simulink model "Motor_Quadcopter_Combined_Current"  (R2016b)
settings: Solver=VariableStepAuto  StartTime=0.0  StopTime=500  RelTol=1e-3
libraries: simulink x36
(part 3 of 5)

== system Motor_Quadcopter_Combined_Current/Nominal/Quadcopter_Arm1/Delta Motor ==
  Vab : Inport
  Vbc : Inport  Port=2
  Vca : Inport  Port=3
  1/Lm : Gain  Gain=100
  1/Lm1 : Gain  Gain=100
  1/Lm2 : Gain  Gain=100
  Add : Sum
  Add1 : Sum
  Constant : Constant  Value=5
  Constant1 : Constant  Value=5
  Constant2 : Constant  Value=5
  Divide : Product  Inputs=*/
  Gain : Gain  Gain=1/3
  Integrator : Integrator
  Integrator1 : Integrator
  Integrator2 : Integrator
  Mux : Mux  Inputs=1
  Product{,1..3} (4 alike) : Product
  motor current : Scope  NumInputPorts=3
  sum{,1..5} (6 alike) : Sum  Inputs=+-
  Out1 : Outport
  Out2 : Outport  Port=2
  wires:
  1/Lm2/1 -> Integrator2/1
  Integrator/1 -> Product1/1, sum5/2, sum3/1
  sum3/1 -> Mux/1, motor current/1  "i1"
  Vab/1 -> sum/1
  Product1/1 -> sum/2
  Integrator1/1 -> sum4/1, sum3/2, Product2/1
  sum1/1 -> 1/Lm1/1
  sum/1 -> 1/Lm/1
  1/Lm1/1 -> Integrator1/1
  Integrator2/1 -> sum5/1, sum4/2, Product3/1
  1/Lm/1 -> Integrator/1
  sum4/1 -> motor current/2  "i2"
  Product2/1 -> sum1/2
  Vca/1 -> sum2/1
  sum5/1 -> motor current/3  "i3"
  sum2/1 -> 1/Lm2/1
  Product3/1 -> sum2/2
  Vbc/1 -> sum1/1
  Mux/1 -> Out1/1
  Product/1 -> Divide/1
  Add/1 -> Divide/2
  Divide/1 -> Add1/1
  Constant/1 -> Add/1, Product/1, Product1/2
  Constant2/1 -> Add1/2, Product3/2
  Constant1/1 -> Add/2, Product/2, Product2/2
  Add1/1 -> Gain/1
  Gain/1 -> Out2/1

== system Motor_Quadcopter_Combined_Current/Nominal/Quadcopter_Arm1/Gate Driver ==
  Relational Operator{1..6} (6 alike) : RelationalOperator  Operator=>  OutDataTypeStr=boolean  RndMeth=Simplest
  Sawtooth{1..6} (6 alike) : SignalGenerator  WaveForm=sawtooth  Frequency=20
  Scope{1..6} (6 alike) : Scope  NumInputPorts=2
  Sine Wave (0 phase) : Sin  Frequency=2*pi  SampleTime=0.001
  Sine Wave (0.5 phase) : Sin  Frequency=2*pi  Phase=0.5*(2*pi)  SampleTime=0.001
  Sine Wave (0.5+1/3 phase) : Sin  Frequency=2*pi  Phase=(0.5 + 1/3)*(2*pi)  SampleTime=0.001
  Sine Wave (0.5+2/3 phase) : Sin  Frequency=2*pi  Phase=(2/3 + 0.5)*2*pi  SampleTime=0.001
  Sine Wave (1/3 phase) : Sin  Frequency=2*pi  Phase=(1/3)*(2*pi)  SampleTime=0.001
  Sine Wave (2/3 phase) : Sin  Frequency=2*pi  Phase=(2/3)*(2*pi)  SampleTime=0.001
  Switch {1..6} (6 alike) : Scope
  Switch 1 PWM : Outport
  Switch 2 PWM : Outport  Port=2
  Switch 3 PWM : Outport  Port=3
  Switch 4 PWM : Outport  Port=4
  Switch 5 PWM : Outport  Port=5
  Switch 6 PWM : Outport  Port=6
  wires:
  Relational Operator4/1 -> Switch 3 PWM/1, Switch 3/1
  Sine Wave (1/3 phase)/1 -> Scope2/1, Relational Operator3/1
  Relational Operator6/1 -> Switch 6 PWM/1, Switch 6/1
  Sine Wave (2/3 phase)/1 -> Scope4/1, Relational Operator4/1
  Sawtooth4/1 -> Scope4/2, Relational Operator4/2
  Sawtooth1/1 -> Scope1/2, Relational Operator1/2
  Relational Operator2/1 -> Switch 5 PWM/1, Switch 5/1
  Sine Wave (0.5+2/3 phase)/1 -> Scope6/1, Relational Operator6/1
  Sawtooth5/1 -> Scope5/2, Relational Operator5/2
  Relational Operator1/1 -> Switch 1 PWM/1, Switch 1/1
  Sawtooth6/1 -> Scope6/2, Relational Operator6/2
  Sine Wave (0 phase)/1 -> Scope1/1, Relational Operator1/1
  Sine Wave (0.5 phase)/1 -> Scope5/1, Relational Operator5/1
  Relational Operator3/1 -> Switch 2 PWM/1, Switch 2/1
  Sine Wave (0.5+1/3 phase)/1 -> Scope3/1, Relational Operator2/1
  Sawtooth2/1 -> Scope3/2, Relational Operator2/2
  Sawtooth3/1 -> Scope2/2, Relational Operator3/2
  Relational Operator5/1 -> Switch 4 PWM/1, Switch 4/1

== system Motor_Quadcopter_Combined_Current/Nominal/Quadcopter_Arm3/Delta Motor ==
  Vab : Inport
  Vbc : Inport  Port=2
  Vca : Inport  Port=3
  1/Lm : Gain  Gain=100
  1/Lm1 : Gain  Gain=100
  1/Lm2 : Gain  Gain=100
  Integrator : Integrator
  Integrator1 : Integrator
  Integrator2 : Integrator
  Rm : Gain  Gain=5
  Rm1 : Gain  Gain=5
  Rm2 : Gain  Gain=5
  motor current : Scope  NumInputPorts=3
  sum{,1..5} (6 alike) : Sum  Inputs=+-
  Out1 : Outport
  wires:
  1/Lm2/1 -> Integrator2/1
  Integrator/1 -> sum5/2, sum3/1, Rm/1
  sum3/1 -> Out1/1, motor current/1  "i1"
  Vab/1 -> sum/1
  Rm/1 -> sum/2
  Integrator1/1 -> sum4/1, sum3/2, Rm1/1
  sum1/1 -> 1/Lm1/1
  sum/1 -> 1/Lm/1
  1/Lm1/1 -> Integrator1/1
  Integrator2/1 -> sum5/1, sum4/2, Rm2/1
  1/Lm/1 -> Integrator/1
  sum4/1 -> motor current/2  "i2"
  Rm1/1 -> sum1/2
  Vca/1 -> sum2/1
  sum5/1 -> motor current/3  "i3"
  sum2/1 -> 1/Lm2/1
  Rm2/1 -> sum2/2
  Vbc/1 -> sum1/1

== system Motor_Quadcopter_Combined_Current/Nominal/Quadcopter_Arm3/Gate Driver ==
  Relational Operator{1..6} (6 alike) : RelationalOperator  Operator=>  OutDataTypeStr=boolean  RndMeth=Simplest
  Sawtooth{1..6} (6 alike) : SignalGenerator  WaveForm=sawtooth  Frequency=20
  Scope{1..6} (6 alike) : Scope  NumInputPorts=2
  Sine Wave (0 phase) : Sin  Frequency=2*pi  SampleTime=0.001
  Sine Wave (0.5 phase) : Sin  Frequency=2*pi  Phase=0.5*(2*pi)  SampleTime=0.001
  Sine Wave (0.5+1/3 phase) : Sin  Frequency=2*pi  Phase=(0.5 + 1/3)*(2*pi)  SampleTime=0.001
  Sine Wave (0.5+2/3 phase) : Sin  Frequency=2*pi  Phase=(2/3 + 0.5)*2*pi  SampleTime=0.001
  Sine Wave (1/3 phase) : Sin  Frequency=2*pi  Phase=(1/3)*(2*pi)  SampleTime=0.001
  Sine Wave (2/3 phase) : Sin  Frequency=2*pi  Phase=(2/3)*(2*pi)  SampleTime=0.001
  Switch {1..6} (6 alike) : Scope
  Switch 1 PWM : Outport
  Switch 2 PWM : Outport  Port=2
  Switch 3 PWM : Outport  Port=3
  Switch 4 PWM : Outport  Port=4
  Switch 5 PWM : Outport  Port=5
  Switch 6 PWM : Outport  Port=6
  wires:
  Relational Operator4/1 -> Switch 3 PWM/1, Switch 3/1
  Sine Wave (1/3 phase)/1 -> Scope2/1, Relational Operator3/1
  Relational Operator6/1 -> Switch 6 PWM/1, Switch 6/1
  Sine Wave (2/3 phase)/1 -> Scope4/1, Relational Operator4/1
  Sawtooth4/1 -> Scope4/2, Relational Operator4/2
  Sawtooth1/1 -> Scope1/2, Relational Operator1/2
  Relational Operator2/1 -> Switch 5 PWM/1, Switch 5/1
  Sine Wave (0.5+2/3 phase)/1 -> Scope6/1, Relational Operator6/1
  Sawtooth5/1 -> Scope5/2, Relational Operator5/2
  Relational Operator1/1 -> Switch 1 PWM/1, Switch 1/1
  Sawtooth6/1 -> Scope6/2, Relational Operator6/2
  Sine Wave (0 phase)/1 -> Scope1/1, Relational Operator1/1
  Sine Wave (0.5 phase)/1 -> Scope5/1, Relational Operator5/1
  Relational Operator3/1 -> Switch 2 PWM/1, Switch 2/1
  Sine Wave (0.5+1/3 phase)/1 -> Scope3/1, Relational Operator2/1
  Sawtooth2/1 -> Scope3/2, Relational Operator2/2
  Sawtooth3/1 -> Scope2/2, Relational Operator3/2
  Relational Operator5/1 -> Switch 4 PWM/1, Switch 4/1

== system Motor_Quadcopter_Combined_Current/Nominal/Quadcopter_Arm4/Delta Motor ==
  Vab : Inport
  Vbc : Inport  Port=2
  Vca : Inport  Port=3
  1/Lm : Gain  Gain=100
  1/Lm1 : Gain  Gain=100
  1/Lm2 : Gain  Gain=100
  Integrator : Integrator
  Integrator1 : Integrator
  Integrator2 : Integrator
  Rm : Gain  Gain=5
  Rm1 : Gain  Gain=5
  Rm2 : Gain  Gain=5
  motor current : Scope  NumInputPorts=3
  sum{,1..5} (6 alike) : Sum  Inputs=+-
  Out1 : Outport
  wires:
  1/Lm2/1 -> Integrator2/1
  Integrator/1 -> sum5/2, sum3/1, Rm/1
  sum3/1 -> Out1/1, motor current/1  "i1"
  Vab/1 -> sum/1
  Rm/1 -> sum/2
  Integrator1/1 -> sum4/1, sum3/2, Rm1/1
  sum1/1 -> 1/Lm1/1
  sum/1 -> 1/Lm/1
  1/Lm1/1 -> Integrator1/1
  Integrator2/1 -> sum5/1, sum4/2, Rm2/1
  1/Lm/1 -> Integrator/1
  sum4/1 -> motor current/2  "i2"
  Rm1/1 -> sum1/2
  Vca/1 -> sum2/1
  sum5/1 -> motor current/3  "i3"
  sum2/1 -> 1/Lm2/1
  Rm2/1 -> sum2/2
  Vbc/1 -> sum1/1

== system Motor_Quadcopter_Combined_Current/Nominal/Quadcopter_Arm4/Gate Driver ==
  Relational Operator{1..6} (6 alike) : RelationalOperator  Operator=>  OutDataTypeStr=boolean  RndMeth=Simplest
  Sawtooth{1..6} (6 alike) : SignalGenerator  WaveForm=sawtooth  Frequency=20
  Scope{1..6} (6 alike) : Scope  NumInputPorts=2
  Sine Wave (0 phase) : Sin  Frequency=2*pi  SampleTime=0.001
  Sine Wave (0.5 phase) : Sin  Frequency=2*pi  Phase=0.5*(2*pi)  SampleTime=0.001
  Sine Wave (0.5+1/3 phase) : Sin  Frequency=2*pi  Phase=(0.5 + 1/3)*(2*pi)  SampleTime=0.001
  Sine Wave (0.5+2/3 phase) : Sin  Frequency=2*pi  Phase=(2/3 + 0.5)*2*pi  SampleTime=0.001
  Sine Wave (1/3 phase) : Sin  Frequency=2*pi  Phase=(1/3)*(2*pi)  SampleTime=0.001
  Sine Wave (2/3 phase) : Sin  Frequency=2*pi  Phase=(2/3)*(2*pi)  SampleTime=0.001
  Switch {1..6} (6 alike) : Scope
  Switch 1 PWM : Outport
  Switch 2 PWM : Outport  Port=2
  Switch 3 PWM : Outport  Port=3
  Switch 4 PWM : Outport  Port=4
  Switch 5 PWM : Outport  Port=5
  Switch 6 PWM : Outport  Port=6
  wires:
  Relational Operator4/1 -> Switch 3 PWM/1, Switch 3/1
  Sine Wave (1/3 phase)/1 -> Scope2/1, Relational Operator3/1
  Relational Operator6/1 -> Switch 6 PWM/1, Switch 6/1
  Sine Wave (2/3 phase)/1 -> Scope4/1, Relational Operator4/1
  Sawtooth4/1 -> Scope4/2, Relational Operator4/2
  Sawtooth1/1 -> Scope1/2, Relational Operator1/2
  Relational Operator2/1 -> Switch 5 PWM/1, Switch 5/1
  Sine Wave (0.5+2/3 phase)/1 -> Scope6/1, Relational Operator6/1
  Sawtooth5/1 -> Scope5/2, Relational Operator5/2
  Relational Operator1/1 -> Switch 1 PWM/1, Switch 1/1
  Sawtooth6/1 -> Scope6/2, Relational Operator6/2
  Sine Wave (0 phase)/1 -> Scope1/1, Relational Operator1/1
  Sine Wave (0.5 phase)/1 -> Scope5/1, Relational Operator5/1
  Relational Operator3/1 -> Switch 2 PWM/1, Switch 2/1
  Sine Wave (0.5+1/3 phase)/1 -> Scope3/1, Relational Operator2/1
  Sawtooth2/1 -> Scope3/2, Relational Operator2/2
  Sawtooth3/1 -> Scope2/2, Relational Operator3/2
  Relational Operator5/1 -> Switch 4 PWM/1, Switch 4/1

== system Motor_Quadcopter_Combined_Current/Nominal/Quatcopter_Arm2/Delta Motor ==
  Vab : Inport
  Vbc : Inport  Port=2
  Vca : Inport  Port=3
  1/Lm : Gain  Gain=100
  1/Lm1 : Gain  Gain=100
  1/Lm2 : Gain  Gain=100
  Integrator : Integrator
  Integrator1 : Integrator
  Integrator2 : Integrator
  Mux : Mux  Inputs=1
  Rm : Gain  Gain=5
  Rm1 : Gain  Gain=5
  Rm2 : Gain  Gain=5
  motor current : Scope  NumInputPorts=3
  sum{,1..5} (6 alike) : Sum  Inputs=+-
  M2_Current : Outport
  wires:
  1/Lm2/1 -> Integrator2/1
  Integrator/1 -> sum5/2, sum3/1, Rm/1
  sum3/1 -> Mux/1, motor current/1  "i1"
  Vab/1 -> sum/1
  Rm/1 -> sum/2
  Integrator1/1 -> sum4/1, sum3/2, Rm1/1
  sum1/1 -> 1/Lm1/1
  sum/1 -> 1/Lm/1
  1/Lm1/1 -> Integrator1/1
  Integrator2/1 -> sum5/1, sum4/2, Rm2/1
  1/Lm/1 -> Integrator/1
  sum4/1 -> motor current/2  "i2"
  Rm1/1 -> sum1/2
  Vca/1 -> sum2/1
  sum5/1 -> motor current/3  "i3"
  sum2/1 -> 1/Lm2/1
  Rm2/1 -> sum2/2
  Vbc/1 -> sum1/1
  Mux/1 -> M2_Current/1

== system Motor_Quadcopter_Combined_Current/Nominal/Quatcopter_Arm2/Gate Driver ==
  Relational Operator{1..6} (6 alike) : RelationalOperator  Operator=>  OutDataTypeStr=boolean  RndMeth=Simplest
  Sawtooth{1..6} (6 alike) : SignalGenerator  WaveForm=sawtooth  Frequency=20
  Scope{1..6} (6 alike) : Scope  NumInputPorts=2
  Sine Wave (0 phase) : Sin  Frequency=2*pi  SampleTime=0.001
  Sine Wave (0.5 phase) : Sin  Frequency=2*pi  Phase=0.5*(2*pi)  SampleTime=0.001
  Sine Wave (0.5+1/3 phase) : Sin  Frequency=2*pi  Phase=(0.5 + 1/3)*(2*pi)  SampleTime=0.001
  Sine Wave (0.5+2/3 phase) : Sin  Frequency=2*pi  Phase=(2/3 + 0.5)*2*pi  SampleTime=0.001
  Sine Wave (1/3 phase) : Sin  Frequency=2*pi  Phase=(1/3)*(2*pi)  SampleTime=0.001
  Sine Wave (2/3 phase) : Sin  Frequency=2*pi  Phase=(2/3)*(2*pi)  SampleTime=0.001
  Switch {1..6} (6 alike) : Scope
  Switch 1 PWM : Outport
  Switch 2 PWM : Outport  Port=2
  Switch 3 PWM : Outport  Port=3
  Switch 4 PWM : Outport  Port=4
  Switch 5 PWM : Outport  Port=5
  Switch 6 PWM : Outport  Port=6
  wires:
  Relational Operator4/1 -> Switch 3 PWM/1, Switch 3/1
  Sine Wave (1/3 phase)/1 -> Scope2/1, Relational Operator3/1
  Relational Operator6/1 -> Switch 6 PWM/1, Switch 6/1
  Sine Wave (2/3 phase)/1 -> Scope4/1, Relational Operator4/1
  Sawtooth4/1 -> Scope4/2, Relational Operator4/2
  Sawtooth1/1 -> Scope1/2, Relational Operator1/2
  Relational Operator2/1 -> Switch 5 PWM/1, Switch 5/1
  Sine Wave (0.5+2/3 phase)/1 -> Scope6/1, Relational Operator6/1
  Sawtooth5/1 -> Scope5/2, Relational Operator5/2
  Relational Operator1/1 -> Switch 1 PWM/1, Switch 1/1
  Sawtooth6/1 -> Scope6/2, Relational Operator6/2
  Sine Wave (0 phase)/1 -> Scope1/1, Relational Operator1/1
  Sine Wave (0.5 phase)/1 -> Scope5/1, Relational Operator5/1
  Relational Operator3/1 -> Switch 2 PWM/1, Switch 2/1
  Sine Wave (0.5+1/3 phase)/1 -> Scope3/1, Relational Operator2/1
  Sawtooth2/1 -> Scope3/2, Relational Operator2/2
  Sawtooth3/1 -> Scope2/2, Relational Operator3/2
  Relational Operator5/1 -> Switch 4 PWM/1, Switch 4/1

== system Motor_Quadcopter_Combined_Current/PWM_Fault/Quadcopter_Arm1/Delta Motor ==
  Vab : Inport
  Vbc : Inport  Port=2
  Vca : Inport  Port=3
  1/Lm : Gain  Gain=100
  1/Lm1 : Gain  Gain=100
  1/Lm2 : Gain  Gain=100
  Add : Sum
  Add1 : Sum
  Constant : Constant  Value=5
  Constant1 : Constant  Value=5
  Constant2 : Constant  Value=5
  Divide : Product  Inputs=*/
  Gain : Gain  Gain=1/3
  Integrator : Integrator
  Integrator1 : Integrator
  Integrator2 : Integrator
  Mux : Mux  Inputs=1
  Product{,1..3} (4 alike) : Product
  motor current : Scope  NumInputPorts=3
  sum{,1..5} (6 alike) : Sum  Inputs=+-
  Out1 : Outport
  Out2 : Outport  Port=2
  wires:
  1/Lm2/1 -> Integrator2/1
  Integrator/1 -> Product1/1, sum5/2, sum3/1
  sum3/1 -> Mux/1, motor current/1  "i1"
  Vab/1 -> sum/1
  Product1/1 -> sum/2
  Integrator1/1 -> sum4/1, sum3/2, Product2/1
  sum1/1 -> 1/Lm1/1
  sum/1 -> 1/Lm/1
  1/Lm1/1 -> Integrator1/1
  Integrator2/1 -> sum5/1, sum4/2, Product3/1
  1/Lm/1 -> Integrator/1
  sum4/1 -> motor current/2  "i2"
  Product2/1 -> sum1/2
  Vca/1 -> sum2/1
  sum5/1 -> motor current/3  "i3"
  sum2/1 -> 1/Lm2/1
  Product3/1 -> sum2/2
  Vbc/1 -> sum1/1
  Mux/1 -> Out1/1
  Product/1 -> Divide/1
  Add/1 -> Divide/2
  Divide/1 -> Add1/1
  Constant/1 -> Add/1, Product/1, Product1/2
  Constant2/1 -> Add1/2, Product3/2
  Constant1/1 -> Add/2, Product/2, Product2/2
  Add1/1 -> Gain/1
  Gain/1 -> Out2/1

== system Motor_Quadcopter_Combined_Current/PWM_Fault/Quadcopter_Arm1/Gate Driver ==
  Relational Operator{1..6} (6 alike) : RelationalOperator  Operator=>  OutDataTypeStr=boolean  RndMeth=Simplest
  Sawtooth{1..6} (6 alike) : SignalGenerator  WaveForm=sawtooth  Frequency=20
  Scope{1..6} (6 alike) : Scope  NumInputPorts=2
  Sine Wave (0 phase) : Sin  Frequency=2*pi  SampleTime=0.001
  Sine Wave (0.5 phase) : Sin  Frequency=2*pi  Phase=0.5*(2*pi)  SampleTime=0.001
  Sine Wave (0.5+1/3 phase) : Sin  Frequency=2*pi  Phase=(0.5 + 1/3)*(2*pi)  SampleTime=0.001
  Sine Wave (0.5+2/3 phase) : Sin  Frequency=2*pi  Phase=(2/3 + 0.5)*2*pi  SampleTime=0.001
  Sine Wave (1/3 phase) : Sin  Frequency=2*pi  Phase=(1/3)*(2*pi)  SampleTime=0.001
  Sine Wave (2/3 phase) : Sin  Frequency=2*pi  Phase=(2/3)*(2*pi)  SampleTime=0.001
  Switch {1..6} (6 alike) : Scope
  Switch 1 PWM : Outport
  Switch 2 PWM : Outport  Port=2
  Switch 3 PWM : Outport  Port=3
  Switch 4 PWM : Outport  Port=4
  Switch 5 PWM : Outport  Port=5
  Switch 6 PWM : Outport  Port=6
  wires:
  Relational Operator4/1 -> Switch 3 PWM/1, Switch 3/1
  Sine Wave (1/3 phase)/1 -> Scope2/1, Relational Operator3/1
  Relational Operator6/1 -> Switch 6 PWM/1, Switch 6/1
  Sine Wave (2/3 phase)/1 -> Scope4/1, Relational Operator4/1
  Sawtooth4/1 -> Scope4/2, Relational Operator4/2
  Sawtooth1/1 -> Scope1/2, Relational Operator1/2
  Relational Operator2/1 -> Switch 5 PWM/1, Switch 5/1
  Sine Wave (0.5+2/3 phase)/1 -> Scope6/1, Relational Operator6/1
  Sawtooth5/1 -> Scope5/2, Relational Operator5/2
  Relational Operator1/1 -> Switch 1 PWM/1, Switch 1/1
  Sawtooth6/1 -> Scope6/2, Relational Operator6/2
  Sine Wave (0 phase)/1 -> Scope1/1, Relational Operator1/1
  Sine Wave (0.5 phase)/1 -> Scope5/1, Relational Operator5/1
  Relational Operator3/1 -> Switch 2 PWM/1, Switch 2/1
  Sine Wave (0.5+1/3 phase)/1 -> Scope3/1, Relational Operator2/1
  Sawtooth2/1 -> Scope3/2, Relational Operator2/2
  Sawtooth3/1 -> Scope2/2, Relational Operator3/2
  Relational Operator5/1 -> Switch 4 PWM/1, Switch 4/1

== system Motor_Quadcopter_Combined_Current/PWM_Fault/Quadcopter_Arm3/Delta Motor ==
  Vab : Inport
  Vbc : Inport  Port=2
  Vca : Inport  Port=3
  1/Lm : Gain  Gain=100
  1/Lm1 : Gain  Gain=100
  1/Lm2 : Gain  Gain=100
  Integrator : Integrator
  Integrator1 : Integrator
  Integrator2 : Integrator
  Rm : Gain  Gain=5
  Rm1 : Gain  Gain=5
  Rm2 : Gain  Gain=5
  motor current : Scope  NumInputPorts=3
  sum{,1..5} (6 alike) : Sum  Inputs=+-
  Out1 : Outport
  wires:
  1/Lm2/1 -> Integrator2/1
  Integrator/1 -> sum5/2, sum3/1, Rm/1
  sum3/1 -> Out1/1, motor current/1  "i1"
  Vab/1 -> sum/1
  Rm/1 -> sum/2
  Integrator1/1 -> sum4/1, sum3/2, Rm1/1
  sum1/1 -> 1/Lm1/1
  sum/1 -> 1/Lm/1
  1/Lm1/1 -> Integrator1/1
  Integrator2/1 -> sum5/1, sum4/2, Rm2/1
  1/Lm/1 -> Integrator/1
  sum4/1 -> motor current/2  "i2"
  Rm1/1 -> sum1/2
  Vca/1 -> sum2/1
  sum5/1 -> motor current/3  "i3"
  sum2/1 -> 1/Lm2/1
  Rm2/1 -> sum2/2
  Vbc/1 -> sum1/1

== system Motor_Quadcopter_Combined_Current/PWM_Fault/Quadcopter_Arm3/Gate Driver ==
  Relational Operator{1..6} (6 alike) : RelationalOperator  Operator=>  OutDataTypeStr=boolean  RndMeth=Simplest
  Sawtooth{1..6} (6 alike) : SignalGenerator  WaveForm=sawtooth  Frequency=20
  Scope{1..6} (6 alike) : Scope  NumInputPorts=2
  Sine Wave (0 phase) : Sin  Frequency=2*pi  SampleTime=0.001
  Sine Wave (0.5 phase) : Sin  Frequency=2*pi  Phase=0.5*(2*pi)  SampleTime=0.001
  Sine Wave (0.5+1/3 phase) : Sin  Frequency=2*pi  Phase=(0.5 + 1/3)*(2*pi)  SampleTime=0.001
  Sine Wave (0.5+2/3 phase) : Sin  Frequency=2*pi  Phase=(2/3 + 0.5)*2*pi  SampleTime=0.001
  Sine Wave (1/3 phase) : Sin  Frequency=2*pi  Phase=(1/3)*(2*pi)  SampleTime=0.001
  Sine Wave (2/3 phase) : Sin  Frequency=2*pi  Phase=(2/3)*(2*pi)  SampleTime=0.001
  Switch {1..6} (6 alike) : Scope
  Switch 1 PWM : Outport
  Switch 2 PWM : Outport  Port=2
  Switch 3 PWM : Outport  Port=3
  Switch 4 PWM : Outport  Port=4
  Switch 5 PWM : Outport  Port=5
  Switch 6 PWM : Outport  Port=6
  wires:
  Relational Operator4/1 -> Switch 3 PWM/1, Switch 3/1
  Sine Wave (1/3 phase)/1 -> Scope2/1, Relational Operator3/1
  Relational Operator6/1 -> Switch 6 PWM/1, Switch 6/1
  Sine Wave (2/3 phase)/1 -> Scope4/1, Relational Operator4/1
  Sawtooth4/1 -> Scope4/2, Relational Operator4/2
  Sawtooth1/1 -> Scope1/2, Relational Operator1/2
  Relational Operator2/1 -> Switch 5 PWM/1, Switch 5/1
  Sine Wave (0.5+2/3 phase)/1 -> Scope6/1, Relational Operator6/1
  Sawtooth5/1 -> Scope5/2, Relational Operator5/2
  Relational Operator1/1 -> Switch 1 PWM/1, Switch 1/1
  Sawtooth6/1 -> Scope6/2, Relational Operator6/2
  Sine Wave (0 phase)/1 -> Scope1/1, Relational Operator1/1
  Sine Wave (0.5 phase)/1 -> Scope5/1, Relational Operator5/1
  Relational Operator3/1 -> Switch 2 PWM/1, Switch 2/1
  Sine Wave (0.5+1/3 phase)/1 -> Scope3/1, Relational Operator2/1
  Sawtooth2/1 -> Scope3/2, Relational Operator2/2
  Sawtooth3/1 -> Scope2/2, Relational Operator3/2
  Relational Operator5/1 -> Switch 4 PWM/1, Switch 4/1

== system Motor_Quadcopter_Combined_Current/PWM_Fault/Quadcopter_Arm4/Delta Motor ==
  Vab : Inport
  Vbc : Inport  Port=2
  Vca : Inport  Port=3
  1/Lm : Gain  Gain=100
  1/Lm1 : Gain  Gain=100
  1/Lm2 : Gain  Gain=100
  Integrator : Integrator
  Integrator1 : Integrator
  Integrator2 : Integrator
  Rm : Gain  Gain=5
  Rm1 : Gain  Gain=5
  Rm2 : Gain  Gain=5
  motor current : Scope  NumInputPorts=3
  sum{,1..5} (6 alike) : Sum  Inputs=+-
  Out1 : Outport
  wires:
  1/Lm2/1 -> Integrator2/1
  Integrator/1 -> sum5/2, sum3/1, Rm/1
  sum3/1 -> Out1/1, motor current/1  "i1"
  Vab/1 -> sum/1
  Rm/1 -> sum/2
  Integrator1/1 -> sum4/1, sum3/2, Rm1/1
  sum1/1 -> 1/Lm1/1
  sum/1 -> 1/Lm/1
  1/Lm1/1 -> Integrator1/1
  Integrator2/1 -> sum5/1, sum4/2, Rm2/1
  1/Lm/1 -> Integrator/1
  sum4/1 -> motor current/2  "i2"
  Rm1/1 -> sum1/2
  Vca/1 -> sum2/1
  sum5/1 -> motor current/3  "i3"
  sum2/1 -> 1/Lm2/1
  Rm2/1 -> sum2/2
  Vbc/1 -> sum1/1

== system Motor_Quadcopter_Combined_Current/PWM_Fault/Quadcopter_Arm4/Gate Driver ==
  Relational Operator{1..6} (6 alike) : RelationalOperator  Operator=>  OutDataTypeStr=boolean  RndMeth=Simplest
  Sawtooth{1..6} (6 alike) : SignalGenerator  WaveForm=sawtooth  Frequency=20
  Scope{1..6} (6 alike) : Scope  NumInputPorts=2
  Sine Wave (0 phase) : Sin  Frequency=2*pi  SampleTime=0.001
  Sine Wave (0.5 phase) : Sin  Frequency=2*pi  Phase=0.5*(2*pi)  SampleTime=0.001
  Sine Wave (0.5+1/3 phase) : Sin  Frequency=2*pi  Phase=(0.5 + 1/3)*(2*pi)  SampleTime=0.001
  Sine Wave (0.5+2/3 phase) : Sin  Frequency=2*pi  Phase=(2/3 + 0.5)*2*pi  SampleTime=0.001
  Sine Wave (1/3 phase) : Sin  Frequency=2*pi  Phase=(1/3)*(2*pi)  SampleTime=0.001
  Sine Wave (2/3 phase) : Sin  Frequency=2*pi  Phase=(2/3)*(2*pi)  SampleTime=0.001
  Switch {1..6} (6 alike) : Scope
  Switch 1 PWM : Outport
  Switch 2 PWM : Outport  Port=2
  Switch 3 PWM : Outport  Port=3
  Switch 4 PWM : Outport  Port=4
  Switch 5 PWM : Outport  Port=5
  Switch 6 PWM : Outport  Port=6
  wires:
  Relational Operator4/1 -> Switch 3 PWM/1, Switch 3/1
  Sine Wave (1/3 phase)/1 -> Scope2/1, Relational Operator3/1
  Relational Operator6/1 -> Switch 6 PWM/1, Switch 6/1
  Sine Wave (2/3 phase)/1 -> Scope4/1, Relational Operator4/1
  Sawtooth4/1 -> Scope4/2, Relational Operator4/2
  Sawtooth1/1 -> Scope1/2, Relational Operator1/2
  Relational Operator2/1 -> Switch 5 PWM/1, Switch 5/1
  Sine Wave (0.5+2/3 phase)/1 -> Scope6/1, Relational Operator6/1
  Sawtooth5/1 -> Scope5/2, Relational Operator5/2
  Relational Operator1/1 -> Switch 1 PWM/1, Switch 1/1
  Sawtooth6/1 -> Scope6/2, Relational Operator6/2
  Sine Wave (0 phase)/1 -> Scope1/1, Relational Operator1/1
  Sine Wave (0.5 phase)/1 -> Scope5/1, Relational Operator5/1
  Relational Operator3/1 -> Switch 2 PWM/1, Switch 2/1
  Sine Wave (0.5+1/3 phase)/1 -> Scope3/1, Relational Operator2/1
  Sawtooth2/1 -> Scope3/2, Relational Operator2/2
  Sawtooth3/1 -> Scope2/2, Relational Operator3/2
  Relational Operator5/1 -> Switch 4 PWM/1, Switch 4/1

== system Motor_Quadcopter_Combined_Current/PWM_Fault/Quatcopter_Arm2/Delta Motor ==
  Vab : Inport
  Vbc : Inport  Port=2
  Vca : Inport  Port=3
  1/Lm : Gain  Gain=100
  1/Lm1 : Gain  Gain=100
  1/Lm2 : Gain  Gain=100
  Integrator : Integrator
  Integrator1 : Integrator
  Integrator2 : Integrator
  Mux : Mux  Inputs=1
  Rm : Gain  Gain=5
  Rm1 : Gain  Gain=5
  Rm2 : Gain  Gain=5
  motor current : Scope  NumInputPorts=3
  sum{,1..5} (6 alike) : Sum  Inputs=+-
  M2_Current : Outport
  wires:
  1/Lm2/1 -> Integrator2/1
  Integrator/1 -> sum5/2, sum3/1, Rm/1
  sum3/1 -> Mux/1, motor current/1  "i1"
  Vab/1 -> sum/1
  Rm/1 -> sum/2
  Integrator1/1 -> sum4/1, sum3/2, Rm1/1
  sum1/1 -> 1/Lm1/1
  sum/1 -> 1/Lm/1
  1/Lm1/1 -> Integrator1/1
  Integrator2/1 -> sum5/1, sum4/2, Rm2/1
  1/Lm/1 -> Integrator/1
  sum4/1 -> motor current/2  "i2"
  Rm1/1 -> sum1/2
  Vca/1 -> sum2/1
  sum5/1 -> motor current/3  "i3"
  sum2/1 -> 1/Lm2/1
  Rm2/1 -> sum2/2
  Vbc/1 -> sum1/1
  Mux/1 -> M2_Current/1

== system Motor_Quadcopter_Combined_Current/PWM_Fault/Quatcopter_Arm2/Gate Driver ==
  Clock : Clock
  Relational Operator{1..6} (6 alike) : RelationalOperator  Operator=>  OutDataTypeStr=boolean  RndMeth=Simplest
  Sawtooth1 : SignalGenerator  WaveForm=sawtooth  Frequency=23
  Sawtooth{2..7} (6 alike) : SignalGenerator  WaveForm=sawtooth  Frequency=20
  Scope{1..6} (6 alike) : Scope  NumInputPorts=2
  Sine Wave (0 phase) : Sin  Frequency=2*pi  SampleTime=0.001
  Sine Wave (0.5 phase) : Sin  Frequency=2*pi  Phase=0.5*(2*pi)  SampleTime=0.001
  Sine Wave (0.5+1/3 phase) : Sin  Frequency=2*pi  Phase=(0.5 + 1/3)*(2*pi)  SampleTime=0.001
  Sine Wave (0.5+2/3 phase) : Sin  Frequency=2*pi  Phase=(2/3 + 0.5)*2*pi  SampleTime=0.001
  Sine Wave (1/3 phase) : Sin  Frequency=2*pi  Phase=(1/3)*(2*pi)  SampleTime=0.001
  Sine Wave (2/3 phase) : Sin  Frequency=2*pi  Phase=(2/3)*(2*pi)  SampleTime=0.001
  Switch : Switch  Threshold=370
  Switch {1..6} (6 alike) : Scope
  Switch 1 PWM : Outport
  Switch 2 PWM : Outport  Port=2
  Switch 3 PWM : Outport  Port=3
  Switch 4 PWM : Outport  Port=4
  Switch 5 PWM : Outport  Port=5
  Switch 6 PWM : Outport  Port=6
  wires:
  Relational Operator4/1 -> Switch 3 PWM/1, Switch 3/1
  Sine Wave (1/3 phase)/1 -> Scope2/1, Relational Operator3/1
  Relational Operator6/1 -> Switch 6 PWM/1, Switch 6/1
  Sine Wave (2/3 phase)/1 -> Scope4/1, Relational Operator4/1
  Sawtooth4/1 -> Scope4/2, Relational Operator4/2
  Relational Operator2/1 -> Switch 5 PWM/1, Switch 5/1
  Sine Wave (0.5+2/3 phase)/1 -> Scope6/1, Relational Operator6/1
  Sawtooth5/1 -> Scope5/2, Relational Operator5/2
  Relational Operator1/1 -> Switch 1 PWM/1, Switch 1/1
  Sawtooth6/1 -> Scope6/2, Relational Operator6/2
  Sine Wave (0 phase)/1 -> Scope1/1, Relational Operator1/1
  Sine Wave (0.5 phase)/1 -> Scope5/1, Relational Operator5/1
  Relational Operator3/1 -> Switch 2 PWM/1, Switch 2/1
  Sine Wave (0.5+1/3 phase)/1 -> Scope3/1, Relational Operator2/1
  Sawtooth2/1 -> Scope3/2, Relational Operator2/2
  Sawtooth3/1 -> Scope2/2, Relational Operator3/2
  Relational Operator5/1 -> Switch 4 PWM/1, Switch 4/1
  Switch/1 -> Scope1/2, Relational Operator1/2
  Sawtooth1/1 -> Switch/1
  Sawtooth7/1 -> Switch/3
  Clock/1 -> Switch/2

== system Motor_Quadcopter_Combined_Current/Stuck_Fault/Quadcopter_Arm1/Delta Motor ==
  Vab : Inport
  Vbc : Inport  Port=2
  Vca : Inport  Port=3
  1/Lm : Gain  Gain=100
  1/Lm1 : Gain  Gain=100
  1/Lm2 : Gain  Gain=100
  Add : Sum
  Add1 : Sum
  Constant : Constant  Value=5
  Constant1 : Constant  Value=5
  Constant2 : Constant  Value=5
  Divide : Product  Inputs=*/
  Gain : Gain  Gain=1/3
  Integrator : Integrator
  Integrator1 : Integrator
  Integrator2 : Integrator
  Mux : Mux  Inputs=1
  Product{,1..3} (4 alike) : Product
  motor current : Scope  NumInputPorts=3
  sum{,1..5} (6 alike) : Sum  Inputs=+-
  Out1 : Outport
  Out2 : Outport  Port=2
  wires:
  1/Lm2/1 -> Integrator2/1
  Integrator/1 -> Product1/1, sum5/2, sum3/1
  sum3/1 -> Mux/1, motor current/1  "i1"
  Vab/1 -> sum/1
  Product1/1 -> sum/2
  Integrator1/1 -> sum4/1, sum3/2, Product2/1
  sum1/1 -> 1/Lm1/1
  sum/1 -> 1/Lm/1
  1/Lm1/1 -> Integrator1/1
  Integrator2/1 -> sum5/1, sum4/2, Product3/1
  1/Lm/1 -> Integrator/1
  sum4/1 -> motor current/2  "i2"
  Product2/1 -> sum1/2
  Vca/1 -> sum2/1
  sum5/1 -> motor current/3  "i3"
  sum2/1 -> 1/Lm2/1
  Product3/1 -> sum2/2
  Vbc/1 -> sum1/1
  Mux/1 -> Out1/1
  Product/1 -> Divide/1
  Add/1 -> Divide/2
  Divide/1 -> Add1/1
  Constant/1 -> Add/1, Product/1, Product1/2
  Constant2/1 -> Add1/2, Product3/2
  Constant1/1 -> Add/2, Product/2, Product2/2
  Add1/1 -> Gain/1
  Gain/1 -> Out2/1

== system Motor_Quadcopter_Combined_Current/Stuck_Fault/Quadcopter_Arm1/Gate Driver ==
  Relational Operator{1..6} (6 alike) : RelationalOperator  Operator=>  OutDataTypeStr=boolean  RndMeth=Simplest
  Sawtooth{1..6} (6 alike) : SignalGenerator  WaveForm=sawtooth  Frequency=20
  Scope{1..6} (6 alike) : Scope  NumInputPorts=2
  Sine Wave (0 phase) : Sin  Frequency=2*pi  SampleTime=0.001
  Sine Wave (0.5 phase) : Sin  Frequency=2*pi  Phase=0.5*(2*pi)  SampleTime=0.001
  Sine Wave (0.5+1/3 phase) : Sin  Frequency=2*pi  Phase=(0.5 + 1/3)*(2*pi)  SampleTime=0.001
  Sine Wave (0.5+2/3 phase) : Sin  Frequency=2*pi  Phase=(2/3 + 0.5)*2*pi  SampleTime=0.001
  Sine Wave (1/3 phase) : Sin  Frequency=2*pi  Phase=(1/3)*(2*pi)  SampleTime=0.001
  Sine Wave (2/3 phase) : Sin  Frequency=2*pi  Phase=(2/3)*(2*pi)  SampleTime=0.001
  Switch {1..6} (6 alike) : Scope
  Switch 1 PWM : Outport
  Switch 2 PWM : Outport  Port=2
  Switch 3 PWM : Outport  Port=3
  Switch 4 PWM : Outport  Port=4
  Switch 5 PWM : Outport  Port=5
  Switch 6 PWM : Outport  Port=6
  wires:
  Relational Operator4/1 -> Switch 3 PWM/1, Switch 3/1
  Sine Wave (1/3 phase)/1 -> Scope2/1, Relational Operator3/1
  Relational Operator6/1 -> Switch 6 PWM/1, Switch 6/1
  Sine Wave (2/3 phase)/1 -> Scope4/1, Relational Operator4/1
  Sawtooth4/1 -> Scope4/2, Relational Operator4/2
  Sawtooth1/1 -> Scope1/2, Relational Operator1/2
  Relational Operator2/1 -> Switch 5 PWM/1, Switch 5/1
  Sine Wave (0.5+2/3 phase)/1 -> Scope6/1, Relational Operator6/1
  Sawtooth5/1 -> Scope5/2, Relational Operator5/2
  Relational Operator1/1 -> Switch 1 PWM/1, Switch 1/1
  Sawtooth6/1 -> Scope6/2, Relational Operator6/2
  Sine Wave (0 phase)/1 -> Scope1/1, Relational Operator1/1
  Sine Wave (0.5 phase)/1 -> Scope5/1, Relational Operator5/1
  Relational Operator3/1 -> Switch 2 PWM/1, Switch 2/1
  Sine Wave (0.5+1/3 phase)/1 -> Scope3/1, Relational Operator2/1
  Sawtooth2/1 -> Scope3/2, Relational Operator2/2
  Sawtooth3/1 -> Scope2/2, Relational Operator3/2
  Relational Operator5/1 -> Switch 4 PWM/1, Switch 4/1

== system Motor_Quadcopter_Combined_Current/Stuck_Fault/Quadcopter_Arm3/Delta Motor ==
  Vab : Inport
  Vbc : Inport  Port=2
  Vca : Inport  Port=3
  1/Lm : Gain  Gain=100
  1/Lm1 : Gain  Gain=100
  1/Lm2 : Gain  Gain=100
  Integrator : Integrator
  Integrator1 : Integrator
  Integrator2 : Integrator
  Rm : Gain  Gain=5
  Rm1 : Gain  Gain=5
  Rm2 : Gain  Gain=5
  motor current : Scope  NumInputPorts=3
  sum{,1..5} (6 alike) : Sum  Inputs=+-
  Out1 : Outport
  wires:
  1/Lm2/1 -> Integrator2/1
  Integrator/1 -> sum5/2, sum3/1, Rm/1
  sum3/1 -> Out1/1, motor current/1  "i1"
  Vab/1 -> sum/1
  Rm/1 -> sum/2
  Integrator1/1 -> sum4/1, sum3/2, Rm1/1
  sum1/1 -> 1/Lm1/1
  sum/1 -> 1/Lm/1
  1/Lm1/1 -> Integrator1/1
  Integrator2/1 -> sum5/1, sum4/2, Rm2/1
  1/Lm/1 -> Integrator/1
  sum4/1 -> motor current/2  "i2"
  Rm1/1 -> sum1/2
  Vca/1 -> sum2/1
  sum5/1 -> motor current/3  "i3"
  sum2/1 -> 1/Lm2/1
  Rm2/1 -> sum2/2
  Vbc/1 -> sum1/1

== system Motor_Quadcopter_Combined_Current/Stuck_Fault/Quadcopter_Arm3/Gate Driver ==
  Relational Operator{1..6} (6 alike) : RelationalOperator  Operator=>  OutDataTypeStr=boolean  RndMeth=Simplest
  Sawtooth{1..6} (6 alike) : SignalGenerator  WaveForm=sawtooth  Frequency=20
  Scope{1..6} (6 alike) : Scope  NumInputPorts=2
  Sine Wave (0 phase) : Sin  Frequency=2*pi  SampleTime=0.001
  Sine Wave (0.5 phase) : Sin  Frequency=2*pi  Phase=0.5*(2*pi)  SampleTime=0.001
  Sine Wave (0.5+1/3 phase) : Sin  Frequency=2*pi  Phase=(0.5 + 1/3)*(2*pi)  SampleTime=0.001
  Sine Wave (0.5+2/3 phase) : Sin  Frequency=2*pi  Phase=(2/3 + 0.5)*2*pi  SampleTime=0.001
  Sine Wave (1/3 phase) : Sin  Frequency=2*pi  Phase=(1/3)*(2*pi)  SampleTime=0.001
  Sine Wave (2/3 phase) : Sin  Frequency=2*pi  Phase=(2/3)*(2*pi)  SampleTime=0.001
  Switch {1..6} (6 alike) : Scope
  Switch 1 PWM : Outport
  Switch 2 PWM : Outport  Port=2
  Switch 3 PWM : Outport  Port=3
  Switch 4 PWM : Outport  Port=4
  Switch 5 PWM : Outport  Port=5
  Switch 6 PWM : Outport  Port=6
  wires:
  Relational Operator4/1 -> Switch 3 PWM/1, Switch 3/1
  Sine Wave (1/3 phase)/1 -> Scope2/1, Relational Operator3/1
  Relational Operator6/1 -> Switch 6 PWM/1, Switch 6/1
  Sine Wave (2/3 phase)/1 -> Scope4/1, Relational Operator4/1
  Sawtooth4/1 -> Scope4/2, Relational Operator4/2
  Sawtooth1/1 -> Scope1/2, Relational Operator1/2
  Relational Operator2/1 -> Switch 5 PWM/1, Switch 5/1
  Sine Wave (0.5+2/3 phase)/1 -> Scope6/1, Relational Operator6/1
  Sawtooth5/1 -> Scope5/2, Relational Operator5/2
  Relational Operator1/1 -> Switch 1 PWM/1, Switch 1/1
  Sawtooth6/1 -> Scope6/2, Relational Operator6/2
  Sine Wave (0 phase)/1 -> Scope1/1, Relational Operator1/1
  Sine Wave (0.5 phase)/1 -> Scope5/1, Relational Operator5/1
  Relational Operator3/1 -> Switch 2 PWM/1, Switch 2/1
  Sine Wave (0.5+1/3 phase)/1 -> Scope3/1, Relational Operator2/1
  Sawtooth2/1 -> Scope3/2, Relational Operator2/2
  Sawtooth3/1 -> Scope2/2, Relational Operator3/2
  Relational Operator5/1 -> Switch 4 PWM/1, Switch 4/1

== system Motor_Quadcopter_Combined_Current/Stuck_Fault/Quadcopter_Arm4/Delta Motor ==
  Vab : Inport
  Vbc : Inport  Port=2
  Vca : Inport  Port=3
  1/Lm : Gain  Gain=100
  1/Lm1 : Gain  Gain=100
  1/Lm2 : Gain  Gain=100
  Add : Sum
  Add1 : Sum
  Constant : Constant  Value=5
  Constant1 : Constant  Value=5
  Constant2 : Constant  Value=5
  Divide : Product  Inputs=*/
  Gain : Gain  Gain=1/3
  Integrator : Integrator
  Integrator1 : Integrator
  Integrator2 : Integrator
  Mux : Mux  Inputs=1
  Product{,1..3} (4 alike) : Product
  motor current : Scope  NumInputPorts=3
  sum{,1..5} (6 alike) : Sum  Inputs=+-
  Out1 : Outport
  Out2 : Outport  Port=2
  wires:
  1/Lm2/1 -> Integrator2/1
  Integrator/1 -> Product1/1, sum5/2, sum3/1
  sum3/1 -> Mux/1, motor current/1  "i1"
  Vab/1 -> sum/1
  Product1/1 -> sum/2
  Integrator1/1 -> sum4/1, sum3/2, Product2/1
  sum1/1 -> 1/Lm1/1
  sum/1 -> 1/Lm/1
  1/Lm1/1 -> Integrator1/1
  Integrator2/1 -> sum5/1, sum4/2, Product3/1
  1/Lm/1 -> Integrator/1
  sum4/1 -> motor current/2  "i2"
  Product2/1 -> sum1/2
  Vca/1 -> sum2/1
  sum5/1 -> motor current/3  "i3"
  sum2/1 -> 1/Lm2/1
  Product3/1 -> sum2/2
  Vbc/1 -> sum1/1
  Mux/1 -> Out1/1
  Product/1 -> Divide/1
  Add/1 -> Divide/2
  Divide/1 -> Add1/1
  Constant/1 -> Add/1, Product/1, Product1/2
  Constant2/1 -> Add1/2, Product3/2
  Constant1/1 -> Add/2, Product/2, Product2/2
  Add1/1 -> Gain/1
  Gain/1 -> Out2/1

== system Motor_Quadcopter_Combined_Current/Stuck_Fault/Quadcopter_Arm4/Gate Driver ==
  Clock : Clock
  Relational Operator{1..6} (6 alike) : RelationalOperator  Operator=>  OutDataTypeStr=boolean  RndMeth=Simplest
  Sawtooth{1..6} (6 alike) : SignalGenerator  WaveForm=sawtooth  Frequency=20
  Sawtooth7 : SignalGenerator  WaveForm=sawtooth  Amplitude=0  Frequency=20
  Scope{1..6} (6 alike) : Scope  NumInputPorts=2
  Sine Wave (0 phase) : Sin  Amplitude=0  Frequency=2*pi  SampleTime=0.001
  Sine Wave (0 phase)1 : Sin  Frequency=2*pi  SampleTime=0.001
  Sine Wave (0.5 phase) : Sin  Frequency=2*pi  Phase=0.5*(2*pi)  SampleTime=0.001
  Sine Wave (0.5+1/3 phase) : Sin  Frequency=2*pi  Phase=(0.5 + 1/3)*(2*pi)  SampleTime=0.001
  Sine Wave (0.5+2/3 phase) : Sin  Frequency=2*pi  Phase=(2/3 + 0.5)*2*pi  SampleTime=0.001
  Sine Wave (1/3 phase) : Sin  Frequency=2*pi  Phase=(1/3)*(2*pi)  SampleTime=0.001
  Sine Wave (2/3 phase) : Sin  Frequency=2*pi  Phase=(2/3)*(2*pi)  SampleTime=0.001
  Switch : Switch  Threshold=325
  Switch {1..6} (6 alike) : Scope
  Switch1 : Switch  Threshold=325
  Switch 1 PWM : Outport
  Switch 2 PWM : Outport  Port=2
  Switch 3 PWM : Outport  Port=3
  Switch 4 PWM : Outport  Port=4
  Switch 5 PWM : Outport  Port=5
  Switch 6 PWM : Outport  Port=6
  wires:
  Relational Operator4/1 -> Switch 3 PWM/1, Switch 3/1
  Sine Wave (1/3 phase)/1 -> Scope2/1, Relational Operator3/1
  Relational Operator6/1 -> Switch 6 PWM/1, Switch 6/1
  Sine Wave (2/3 phase)/1 -> Scope4/1, Relational Operator4/1
  Sawtooth4/1 -> Scope4/2, Relational Operator4/2
  Relational Operator2/1 -> Switch 5 PWM/1, Switch 5/1
  Sine Wave (0.5+2/3 phase)/1 -> Scope6/1, Relational Operator6/1
  Sawtooth5/1 -> Scope5/2, Relational Operator5/2
  Relational Operator1/1 -> Switch 1 PWM/1, Switch 1/1
  Sawtooth6/1 -> Scope6/2, Relational Operator6/2
  Sine Wave (0.5 phase)/1 -> Scope5/1, Relational Operator5/1
  Relational Operator3/1 -> Switch 2 PWM/1, Switch 2/1
  Sine Wave (0.5+1/3 phase)/1 -> Scope3/1, Relational Operator2/1
  Sawtooth2/1 -> Scope3/2, Relational Operator2/2
  Sawtooth3/1 -> Scope2/2, Relational Operator3/2
  Relational Operator5/1 -> Switch 4 PWM/1, Switch 4/1
  Switch/1 -> Scope1/1, Relational Operator1/1
  Clock/1 -> Switch1/2, Switch/2
  Sine Wave (0 phase)/1 -> Switch/1
  Sine Wave (0 phase)1/1 -> Switch/3
  Sawtooth7/1 -> Switch1/1
  Sawtooth1/1 -> Switch1/3
  Switch1/1 -> Relational Operator1/2, Scope1/2

== system Motor_Quadcopter_Combined_Current/Stuck_Fault/Quatcopter_Arm2/Delta Motor ==
  Vab : Inport
  Vbc : Inport  Port=2
  Vca : Inport  Port=3
  1/Lm : Gain  Gain=100
  1/Lm1 : Gain  Gain=100
  1/Lm2 : Gain  Gain=100
  Integrator : Integrator
  Integrator1 : Integrator
  Integrator2 : Integrator
  Mux : Mux  Inputs=1
  Rm : Gain  Gain=5
  Rm1 : Gain  Gain=5
  Rm2 : Gain  Gain=5
  motor current : Scope  NumInputPorts=3
  sum{,1..5} (6 alike) : Sum  Inputs=+-
  M2_Current : Outport
  wires:
  1/Lm2/1 -> Integrator2/1
  Integrator/1 -> sum5/2, sum3/1, Rm/1
  sum3/1 -> Mux/1, motor current/1  "i1"
  Vab/1 -> sum/1
  Rm/1 -> sum/2
  Integrator1/1 -> sum4/1, sum3/2, Rm1/1
  sum1/1 -> 1/Lm1/1
  sum/1 -> 1/Lm/1
  1/Lm1/1 -> Integrator1/1
  Integrator2/1 -> sum5/1, sum4/2, Rm2/1
  1/Lm/1 -> Integrator/1
  sum4/1 -> motor current/2  "i2"
  Rm1/1 -> sum1/2
  Vca/1 -> sum2/1
  sum5/1 -> motor current/3  "i3"
  sum2/1 -> 1/Lm2/1
  Rm2/1 -> sum2/2
  Vbc/1 -> sum1/1
  Mux/1 -> M2_Current/1

== system Motor_Quadcopter_Combined_Current/Stuck_Fault/Quatcopter_Arm2/Gate Driver ==
  Relational Operator{1..6} (6 alike) : RelationalOperator  Operator=>  OutDataTypeStr=boolean  RndMeth=Simplest
  Sawtooth{1..6} (6 alike) : SignalGenerator  WaveForm=sawtooth  Frequency=20
  Scope{1..6} (6 alike) : Scope  NumInputPorts=2
  Sine Wave (0 phase) : Sin  Frequency=2*pi  SampleTime=0.001
  Sine Wave (0.5 phase) : Sin  Frequency=2*pi  Phase=0.5*(2*pi)  SampleTime=0.001
  Sine Wave (0.5+1/3 phase) : Sin  Frequency=2*pi  Phase=(0.5 + 1/3)*(2*pi)  SampleTime=0.001
  Sine Wave (0.5+2/3 phase) : Sin  Frequency=2*pi  Phase=(2/3 + 0.5)*2*pi  SampleTime=0.001
  Sine Wave (1/3 phase) : Sin  Frequency=2*pi  Phase=(1/3)*(2*pi)  SampleTime=0.001
  Sine Wave (2/3 phase) : Sin  Frequency=2*pi  Phase=(2/3)*(2*pi)  SampleTime=0.001
  Switch {1..6} (6 alike) : Scope
  Switch 1 PWM : Outport
  Switch 2 PWM : Outport  Port=2
  Switch 3 PWM : Outport  Port=3
  Switch 4 PWM : Outport  Port=4
  Switch 5 PWM : Outport  Port=5
  Switch 6 PWM : Outport  Port=6
  wires:
  Relational Operator4/1 -> Switch 3 PWM/1, Switch 3/1
  Sine Wave (1/3 phase)/1 -> Scope2/1, Relational Operator3/1
  Relational Operator6/1 -> Switch 6 PWM/1, Switch 6/1
  Sine Wave (2/3 phase)/1 -> Scope4/1, Relational Operator4/1
  Sawtooth4/1 -> Scope4/2, Relational Operator4/2
  Sawtooth1/1 -> Scope1/2, Relational Operator1/2
  Relational Operator2/1 -> Switch 5 PWM/1, Switch 5/1
  Sine Wave (0.5+2/3 phase)/1 -> Scope6/1, Relational Operator6/1
  Sawtooth5/1 -> Scope5/2, Relational Operator5/2
  Relational Operator1/1 -> Switch 1 PWM/1, Switch 1/1
  Sawtooth6/1 -> Scope6/2, Relational Operator6/2
  Sine Wave (0 phase)/1 -> Scope1/1, Relational Operator1/1
  Sine Wave (0.5 phase)/1 -> Scope5/1, Relational Operator5/1
  Relational Operator3/1 -> Switch 2 PWM/1, Switch 2/1
  Sine Wave (0.5+1/3 phase)/1 -> Scope3/1, Relational Operator2/1
  Sawtooth2/1 -> Scope3/2, Relational Operator2/2
  Sawtooth3/1 -> Scope2/2, Relational Operator3/2
  Relational Operator5/1 -> Switch 4 PWM/1, Switch 4/1

== matlab function Motor_Quadcopter_Combined_Current/Nominal/Quatcopter_Arm2/Working MOSFET1 ==
  data: Vds input; Vgs input; R input; K input; Vth input; Vout output
function Vout   = MOSFET(Vds, Vgs, R, K, Vth)
Ids = 0;
Vd = 0;

    % if gate-source voltage does not exceed threshold, switch is open
    % no current through
    if Vgs <= Vth
        Vd = 0;
        Ids = 0;
        
    % if MOSFET is in linear region    
    elseif Vds<(Vgs-Vth)
        Vd = 20;
        Ids = K*(((Vgs - Vth)*Vds)-((Vds^2)/2));
        
     % if MOSFET is in saturation region   
    elseif (Vgs-Vth)<Vds
         Vd = 20;
         Ids = (K/2)*((Vgs-Vth)^2);         
    end

%calculate voltage output
%this voltage goes to the motor
Vout = Vd - Ids*R;

== matlab function Motor_Quadcopter_Combined_Current/Nominal/Quadcopter_Arm1/Working MOSFET2 ==
  data: Vds input; Vgs input; R input; K input; Vth input; Vout output
function Vout   = MOSFET(Vds, Vgs, R, K, Vth)
Ids = 0;
Vd = 0;

    % if gate-source voltage does not exceed threshold, switch is open
    % no current through
    if Vgs <= Vth
        Vd = 0;
        Ids = 0;
        
    % if MOSFET is in linear region    
    elseif Vds<(Vgs-Vth)
        Vd = 20;
        Ids = K*(((Vgs - Vth)*Vds)-((Vds^2)/2));
        
     % if MOSFET is in saturation region   
    elseif (Vgs-Vth)<Vds
         Vd = 20;
         Ids = (K/2)*((Vgs-Vth)^2);         
    end

%calculate voltage output
%this voltage goes to the motor
Vout = Vd - Ids*R;

== matlab function Motor_Quadcopter_Combined_Current/Nominal/Quadcopter_Arm1/Working MOSFET3 ==
  data: Vds input; Vgs input; R input; K input; Vth input; Vout output
function Vout   = MOSFET(Vds, Vgs, R, K, Vth)
Ids = 0;
Vd = 0;

    % if gate-source voltage does not exceed threshold, switch is open
    % no current through
    if Vgs <= Vth
        Vd = 0;
        Ids = 0;
        
    % if MOSFET is in linear region    
    elseif Vds<(Vgs-Vth)
        Vd = 20;
        Ids = K*(((Vgs - Vth)*Vds)-((Vds^2)/2));
        
     % if MOSFET is in saturation region   
    elseif (Vgs-Vth)<Vds
         Vd = 20;
         Ids = (K/2)*((Vgs-Vth)^2);         
    end

%calculate voltage output
%this voltage goes to the motor
Vout = Vd - Ids*R;

== matlab function Motor_Quadcopter_Combined_Current/Nominal/Quadcopter_Arm1/Working MOSFET4 ==
  data: Vds input; Vgs input; R input; K input; Vth input; Vout output
function Vout   = MOSFET(Vds, Vgs, R, K, Vth)
Ids = 0;
Vd = 0;

    % if gate-source voltage does not exceed threshold, switch is open
    % no current through
    if Vgs <= Vth
        Vd = 0;
        Ids = 0;
        
    % if MOSFET is in linear region    
    elseif Vds<(Vgs-Vth)
        Vd = 20;
        Ids = K*(((Vgs - Vth)*Vds)-((Vds^2)/2));
        
     % if MOSFET is in saturation region   
    elseif (Vgs-Vth)<Vds
         Vd = 20;
         Ids = (K/2)*((Vgs-Vth)^2);         
    end

%calculate voltage output
%this voltage goes to the motor
Vout = Vd - Ids*R;

== matlab function Motor_Quadcopter_Combined_Current/Nominal/Quadcopter_Arm1/Working MOSFET5 ==
  data: Vds input; Vgs input; R input; K input; Vth input; Vout output
function Vout   = MOSFET(Vds, Vgs, R, K, Vth)
Ids = 0;
Vd = 0;

    % if gate-source voltage does not exceed threshold, switch is open
    % no current through
    if Vgs <= Vth
        Vd = 0;
        Ids = 0;
        
    % if MOSFET is in linear region    
    elseif Vds<(Vgs-Vth)
        Vd = 20;
        Ids = K*(((Vgs - Vth)*Vds)-((Vds^2)/2));
        
     % if MOSFET is in saturation region   
    elseif (Vgs-Vth)<Vds
         Vd = 20;
         Ids = (K/2)*((Vgs-Vth)^2);         
    end

%calculate voltage output
%this voltage goes to the motor
Vout = Vd - Ids*R;

== matlab function Motor_Quadcopter_Combined_Current/Nominal/Quadcopter_Arm1/Working MOSFET6 ==
  data: Vds input; Vgs input; R input; K input; Vth input; Vout output
function Vout   = MOSFET(Vds, Vgs, R, K, Vth)
Ids = 0;
Vd = 0;

    % if gate-source voltage does not exceed threshold, switch is open
    % no current through
    if Vgs <= Vth
        Vd = 0;
        Ids = 0;
        
    % if MOSFET is in linear region    
    elseif Vds<(Vgs-Vth)
        Vd = 20;
        Ids = K*(((Vgs - Vth)*Vds)-((Vds^2)/2));
        
     % if MOSFET is in saturation region   
    elseif (Vgs-Vth)<Vds
         Vd = 20;
         Ids = (K/2)*((Vgs-Vth)^2);         
    end

%calculate voltage output
%this voltage goes to the motor
Vout = Vd - Ids*R;

== matlab function Motor_Quadcopter_Combined_Current/Nominal/Quatcopter_Arm2/Working MOSFET2 ==
  data: Vds input; Vgs input; R input; K input; Vth input; Vout output
function Vout   = MOSFET(Vds, Vgs, R, K, Vth)
Ids = 0;
Vd = 0;

    % if gate-source voltage does not exceed threshold, switch is open
    % no current through
    if Vgs <= Vth
        Vd = 0;
        Ids = 0;
        
    % if MOSFET is in linear region    
    elseif Vds<(Vgs-Vth)
        Vd = 20;
        Ids = K*(((Vgs - Vth)*Vds)-((Vds^2)/2));
        
     % if MOSFET is in saturation region   
    elseif (Vgs-Vth)<Vds
         Vd = 20;
         Ids = (K/2)*((Vgs-Vth)^2);         
    end

%calculate voltage output
%this voltage goes to the motor
Vout = Vd - Ids*R;

== matlab function Motor_Quadcopter_Combined_Current/Nominal/Quatcopter_Arm2/Working MOSFET3 ==
  data: Vds input; Vgs input; R input; K input; Vth input; Vout output
function Vout   = MOSFET(Vds, Vgs, R, K, Vth)
Ids = 0;
Vd = 0;

    % if gate-source voltage does not exceed threshold, switch is open
    % no current through
    if Vgs <= Vth
        Vd = 0;
        Ids = 0;
        
    % if MOSFET is in linear region    
    elseif Vds<(Vgs-Vth)
        Vd = 20;
        Ids = K*(((Vgs - Vth)*Vds)-((Vds^2)/2));
        
     % if MOSFET is in saturation region   
    elseif (Vgs-Vth)<Vds
         Vd = 20;
         Ids = (K/2)*((Vgs-Vth)^2);         
    end

%calculate voltage output
%this voltage goes to the motor
Vout = Vd - Ids*R;

== matlab function Motor_Quadcopter_Combined_Current/Nominal/Quadcopter_Arm1/Working MOSFET1 ==
  data: Vds input; Vgs input; R input; K input; Vth input; Vout output
function Vout   = MOSFET(Vds, Vgs, R, K, Vth)
Ids = 0;
Vd = 0;

    % if gate-source voltage does not exceed threshold, switch is open
    % no current through
    if Vgs <= Vth
        Vd = 0;
        Ids = 0;
        
    % if MOSFET is in linear region    
    elseif Vds<(Vgs-Vth)
        Vd = 20;
        Ids = K*(((Vgs - Vth)*Vds)-((Vds^2)/2));
        
     % if MOSFET is in saturation region   
    elseif (Vgs-Vth)<Vds
         Vd = 20;
         Ids = (K/2)*((Vgs-Vth)^2);         
    end

%calculate voltage output
%this voltage goes to the motor
Vout = Vd - Ids*R;

== matlab function Motor_Quadcopter_Combined_Current/Nominal/Quatcopter_Arm2/Working MOSFET4 ==
  data: Vds input; Vgs input; R input; K input; Vth input; Vout output
function Vout   = MOSFET(Vds, Vgs, R, K, Vth)
Ids = 0;
Vd = 0;

    % if gate-source voltage does not exceed threshold, switch is open
    % no current through
    if Vgs <= Vth
        Vd = 0;
        Ids = 0;
        
    % if MOSFET is in linear region    
    elseif Vds<(Vgs-Vth)
        Vd = 20;
        Ids = K*(((Vgs - Vth)*Vds)-((Vds^2)/2));
        
     % if MOSFET is in saturation region   
    elseif (Vgs-Vth)<Vds
         Vd = 20;
         Ids = (K/2)*((Vgs-Vth)^2);         
    end

%calculate voltage output
%this voltage goes to the motor
Vout = Vd - Ids*R;

== matlab function Motor_Quadcopter_Combined_Current/Nominal/Quatcopter_Arm2/Working MOSFET5 ==
  data: Vds input; Vgs input; R input; K input; Vth input; Vout output
function Vout   = MOSFET(Vds, Vgs, R, K, Vth)
Ids = 0;
Vd = 0;

    % if gate-source voltage does not exceed threshold, switch is open
    % no current through
    if Vgs <= Vth
        Vd = 0;
        Ids = 0;
        
    % if MOSFET is in linear region    
    elseif Vds<(Vgs-Vth)
        Vd = 20;
        Ids = K*(((Vgs - Vth)*Vds)-((Vds^2)/2));
        
     % if MOSFET is in saturation region   
    elseif (Vgs-Vth)<Vds
         Vd = 20;
         Ids = (K/2)*((Vgs-Vth)^2);         
    end

%calculate voltage output
%this voltage goes to the motor
Vout = Vd - Ids*R;

== matlab function Motor_Quadcopter_Combined_Current/Nominal/Quatcopter_Arm2/Working MOSFET6 ==
  data: Vds input; Vgs input; R input; K input; Vth input; Vout output
function Vout   = MOSFET(Vds, Vgs, R, K, Vth)
Ids = 0;
Vd = 0;

    % if gate-source voltage does not exceed threshold, switch is open
    % no current through
    if Vgs <= Vth
        Vd = 0;
        Ids = 0;
        
    % if MOSFET is in linear region    
    elseif Vds<(Vgs-Vth)
        Vd = 20;
        Ids = K*(((Vgs - Vth)*Vds)-((Vds^2)/2));
        
     % if MOSFET is in saturation region   
    elseif (Vgs-Vth)<Vds
         Vd = 20;
         Ids = (K/2)*((Vgs-Vth)^2);         
    end

%calculate voltage output
%this voltage goes to the motor
Vout = Vd - Ids*R;

== matlab function Motor_Quadcopter_Combined_Current/Nominal/Quadcopter_Arm3/Working MOSFET1 ==
  data: Vds input; Vgs input; R input; K input; Vth input; Vout output
function Vout   = MOSFET(Vds, Vgs, R, K, Vth)
Ids = 0;
Vd = 0;

    % if gate-source voltage does not exceed threshold, switch is open
    % no current through
    if Vgs <= Vth
        Vd = 0;
        Ids = 0;
        
    % if MOSFET is in linear region    
    elseif Vds<(Vgs-Vth)
        Vd = 20;
        Ids = K*(((Vgs - Vth)*Vds)-((Vds^2)/2));
        
     % if MOSFET is in saturation region   
    elseif (Vgs-Vth)<Vds
         Vd = 20;
         Ids = (K/2)*((Vgs-Vth)^2);         
    end

%calculate voltage output
%this voltage goes to the motor
Vout = Vd - Ids*R;

== matlab function Motor_Quadcopter_Combined_Current/Nominal/Quadcopter_Arm3/Working MOSFET2 ==
  data: Vds input; Vgs input; R input; K input; Vth input; Vout output
function Vout   = MOSFET(Vds, Vgs, R, K, Vth)
Ids = 0;
Vd = 0;

    % if gate-source voltage does not exceed threshold, switch is open
    % no current through
    if Vgs <= Vth
        Vd = 0;
        Ids = 0;
        
    % if MOSFET is in linear region    
    elseif Vds<(Vgs-Vth)
        Vd = 20;
        Ids = K*(((Vgs - Vth)*Vds)-((Vds^2)/2));
        
     % if MOSFET is in saturation region   
    elseif (Vgs-Vth)<Vds
         Vd = 20;
         Ids = (K/2)*((Vgs-Vth)^2);         
    end

%calculate voltage output
%this voltage goes to the motor
Vout = Vd - Ids*R;
